simulink model "stateflow_box"  (R2015b)
settings: Solver=VariableStepAuto  StartTime=0.0  StopTime=10.0  RelTol=1e-3
settings Model: Creator=ladmin  LastModifiedBy=ladmin

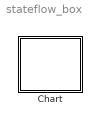
== system stateflow_box ==
  Chart : Stateflow chart  TreatAsAtomicUnit=on

== stateflow chart stateflow_box/Chart ==
  state Box with bigger font [group]
  state Simple Box [group]
